simulink model "One_Meter"  (R2022a)
settings: Solver=FixedStepDiscrete  StartTime=0.0  StopTime=10  FixedStep=0.01  RelTol=1e-3
undefined symbols (not defined in the file): InputPWM, ticksPerRot, Ts, wheelR, WheelSpeed
libraries: mobileRoboticsTrainingLib x5, slpidlib x1
settings Model: Creator=Admin  LastModifiedBy=sarah

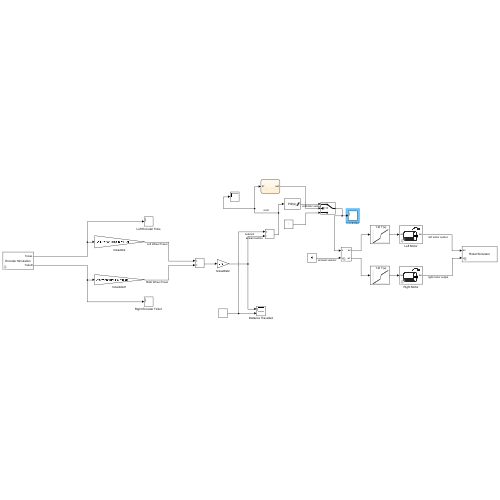
[thumbnail: Simulink's stored preview of the top-level diagram]
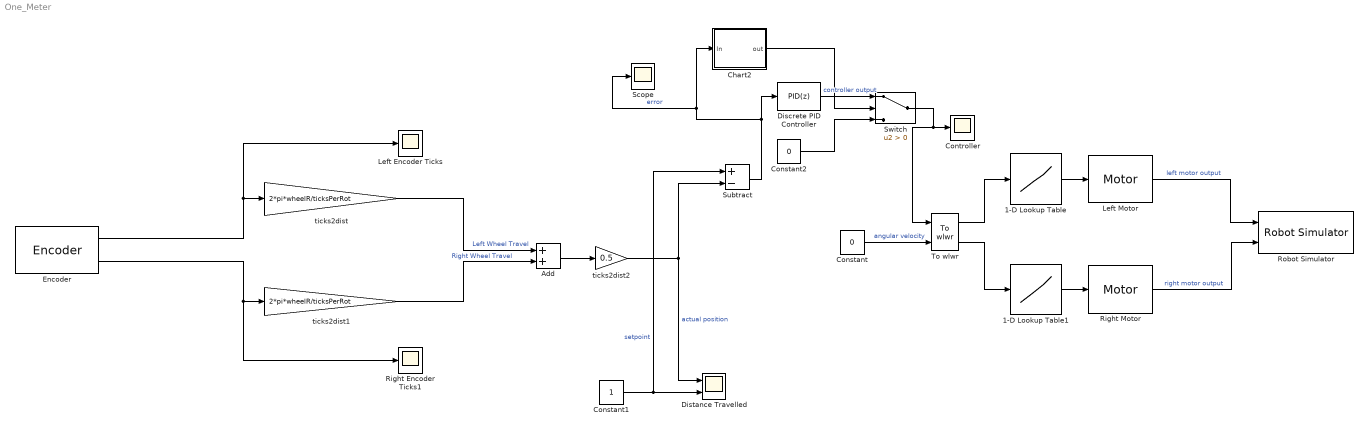
== system One_Meter ==
  1-D Lookup Table : Lookup_n-D  NumberOfTableDimensions=1  BreakpointsForDimension1=WheelSpeed  Table=InputPWM  InternalRulePriority=Speed  RndMeth=Simplest
  1-D Lookup Table1 : Lookup_n-D  NumberOfTableDimensions=1  BreakpointsForDimension1=WheelSpeed  Table=InputPWM  InternalRulePriority=Speed  RndMeth=Simplest
  Add : Sum
  Chart2 : Stateflow chart  TreatAsAtomicUnit=on
  Constant : Constant  Value=0
  Constant1 : Constant
  Constant2 : Constant  Value=0
  Controller : Scope
  Discrete PID Controller : slpidlib/PID Controller  Controller=PID  Form=Parallel  TimeDomain=Discrete-time  UseExternalTs=off  SampleTime=Ts  IntegratorMethod=Forward Euler  FilterMethod=Forward Euler  ControllerParametersSource=internal  P=1.5096  I=0.25346  UseKiTs=off  D=0.40505  N=18.3209  UseFilter=on  TunerSelectOption=Transfer Function Based (PID Tuner App)  InitialConditionSource=internal  InitialConditionForIntegrator=0  InitialConditionForFilter=0  DifferentiatorICPrevScaledInput=0  ExternalReset=none  TrackingMode=off  Kt=1  LimitOutput=on  SatLimitsSource=internal  UpperSaturationLimit=0.52  LowerSaturationLimit=-0.52  LinearizeAsGain=off  AntiWindupMode=clamping  Kb=1  POutMin=[]  POutMax=[]  IOutMin=[]  IOutMax=[]  DOutMin=[]  DOutMax=[]  NOutMin=[]  NOutMax=[]  SumOutMin=[]  SumOutMax=[]  SaturationOutMin=[]  SaturationOutMax=[]  PParamMin=[]  PParamMax=[]  IParamMin=[]  IParamMax=[]  DParamMin=[]  DParamMax=[]  NParamMin=[]  NParamMax=[]  KbParamMin=[]  KbParamMax=[]  KtParamMin=[]  KtParamMax=[]  KbOutMin=[]  KbOutMax=[]  KtOutMin=[]  KtOutMax=[]  IntegratorOutMin=[]  IntegratorOutMax=[]  FilterOutMin=[]  FilterOutMax=[]  SumI1OutMin=[]  SumI1OutMax=[]  SumI2OutMin=[]  SumI2OutMax=[]  SumI3OutMin=[]  SumI3OutMax=[]  SumI4OutMin=[]  SumI4OutMax=[]  SumDOutMin=[]  SumDOutMax=[]  DifferentiatorOutMin=[]  DifferentiatorOutMax=[]  FilterDiffOutCoefMin=[]  FilterDiffOutCoefMax=[]  ReciprocalOutMin=[]  ReciprocalOutMax=[]  SumDenOutMin=[]  SumDenOutMax=[]  SumNumOutMin=[]  SumNumOutMax=[]  DivideOutMin=[]  DivideOutMax=[]  UdiffTsProdOutMin=[]  UdiffTsProdOutMax=[]  NTsProdOutMin=[]  NTsProdOutMax=[]  UintegralTsProdOutMin=[]  UintegralTsProdOutMax=[]  UngainTsProdOutMin=[]  UngainTsProdOutMax=[]  IntegratorContinuousStateAttributes=''  IntegratorStateMustResolveToSignalObject=off  IntegratorRTWStateStorageClass=Auto  FilterContinuousStateAttributes=''  FilterStateMustResolveToSignalObject=off  FilterRTWStateStorageClass=Auto  ParallelPVariant=InternalParameters  IdealPVariant=Disabled  IVariant=InternalParameters  DVariant=InternalParameters  IntegratorVariant=Discrete  SatVariant=Enabled  AWVariant=DiscClampingParallel  PCopyVariant=Disabled  TRVariant=Disabled  FdbkBlocksVariant=Forward  IdealPFdbkVariant=Disabled  SatFdbkVariant=Disabled  DerivativeFilterVariant=ForwardEulerFilter  NVariant=InternalParameters  NCopyVariant=Disabled  FilterICVariant=InternalICsFilter  IntegratorICVariant=InternalICs  ExternalResetVariant=Disabled  TRSumVariant=Passthrough  SumFdbkVariant=Disabled  SumVariant=Sum_PID  TsampFilterVariant=InternalTs  TsampNgainVariant=Passthrough  TsampIntegralVariant=Passthrough  ExternalSaturationOutDataTypeStr=Inherit: Same as second input  aMode=0
  Distance Travelled : Scope  NumInputPorts=2
  Encoder : mobileRoboticsTrainingLib/Encoder  axleLength=axleLength  wheelR=wheelR  ticksPerRot=ticksPerRot
      settings: SourceProductName=Mobile Robotics Training Library
  Left Encoder Ticks : Scope
  Left Motor : mobileRoboticsTrainingLib/Motor  motorPlant=wheelMotorModel  sensorType=Speed
      settings: SourceProductName=Mobile Robotics Training Library
  Right Encoder Ticks1 : Scope
  Right Motor : mobileRoboticsTrainingLib/Motor  motorPlant=wheelMotorModel  sensorType=Speed
      settings: SourceProductName=Mobile Robotics Training Library
  Robot Simulator : mobileRoboticsTrainingLib/Robot Simulator  Priority=99  mapVar=[]  startX=1  startY=1  startTheta=0  axleLength=axleLength  wheelR=wheelR
  Scope : Scope
  Subtract : Sum  Inputs=+-
  Switch : Switch  Criteria=u2 > Threshold  SaturateOnIntegerOverflow=off  InputSameDT=off
  To wlwr : mobileRoboticsTrainingLib/To wlwr  axleLength=axleLength  wheelR=wheelR
  ticks2dist : Gain  Gain=2*pi*wheelR/ticksPerRot
  ticks2dist1 : Gain  Gain=2*pi*wheelR/ticksPerRot
  ticks2dist2 : Gain  Gain=0.5
  wires:
  Encoder/1 -> ticks2dist/1, Left Encoder Ticks/1
  ticks2dist/1 -> Add/1  "Left Wheel Travel"
  Encoder/2 -> Right Encoder Ticks1/1, ticks2dist1/1
  ticks2dist1/1 -> Add/2  "Right Wheel Travel"
  Add/1 -> ticks2dist2/1
  ticks2dist2/1 -> Subtract/2, Distance Travelled/1  "actual position"
  Constant/1 -> To wlwr/2  "angular velocity"
  1-D Lookup Table/1 -> Left Motor/1
  To wlwr/1 -> 1-D Lookup Table/1
  Left Motor/1 -> Robot Simulator/1  "left motor output"
  1-D Lookup Table1/1 -> Right Motor/1
  To wlwr/2 -> 1-D Lookup Table1/1
  Right Motor/1 -> Robot Simulator/2  "right motor output"
  Constant1/1 -> Subtract/1, Distance Travelled/2  "setpoint"
  Subtract/1 -> Discrete PID Controller/1, Chart2/1(In), Scope/1  "error"
  Chart2/1(out) -> Switch/2
  Constant2/1 -> Switch/3
  Discrete PID Controller/1 -> Switch/1  "controller output"
  Switch/1 -> To wlwr/1, Controller/1

== stateflow chart One_Meter/Chart2 ==
  state moving
    entry:
    out = 1;
  state stop
    entry:
    out = 0;
  (default) -> moving
  moving -> stop : [In < 0]
  data: out output; In input
